simulink model "PushPullDCACConverter"  (R2018a)
settings: Solver=VariableStepAuto  StartTime=0.0  StopTime=0.3  RelTol=1e-3
libraries: powerlib x7, powerlib_meascontrol x1
settings Model: Creator=Rodney Tan  LastModifiedBy=Rodney Tan

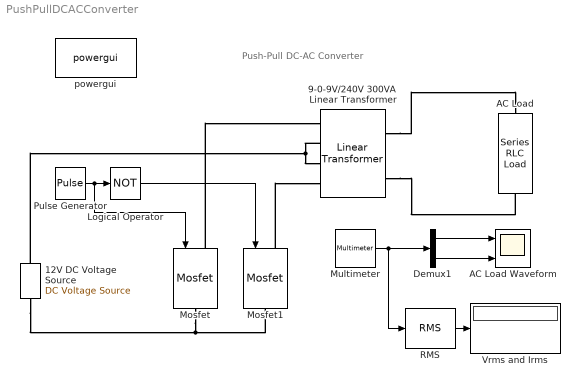
== system PushPullDCACConverter ==
  note: Push-Pull DC-AC Converter
  12V DC Voltage Source : powerlib/Electrical Sources/DC Voltage Source  Amplitude=12  Measurements=None
  9-0-9V/240V 300VA Linear Transformer : powerlib/Elements/Linear Transformer  UNITS=pu  NominalPower=[ 300 50 ]  winding1="[ 240  0.002  0.08 ]"  winding2="[ 9  0.002  0.08 ]"  ThreeWindings=on  winding3=[ 9 0.002 0.08 ]  RmLm=[ 500 500 ]  Measurements=None  DataType=off
  AC Load : powerlib/Elements/Series RLC Load  LConnTagsString=a  RConnTagsString=__new0  NominalVoltage=240  NominalFrequency=50  ActivePower=250  InductivePower=0  CapacitivePower=0  Setx0=off  InitialVoltage=0  SetiL0=off  InitialCurrent=0  Measurements=Branch voltage and current  LoadType=constant Z
  AC Load Waveform : Scope  NumInputPorts=2
  Demux1 : Demux  Outputs=2
  Logical Operator : Logic  Operator=NOT  AllPortsSameDT=off  OutDataTypeStr=boolean
  Mosfet : powerlib/Power Electronics/Mosfet  Ron=0.1  Lon=0  Rd=0.01  Vfd=0  IC=0  Rs=1e5  Cs=inf  Measurements=off
  Mosfet1 : powerlib/Power Electronics/Mosfet  Ron=0.1  Lon=0  Rd=0.01  Vfd=0  IC=0  Rs=1e5  Cs=inf  Measurements=off
  Multimeter : powerlib/Measurements/Multimeter  PhasorSimulation=off  OutputType=Complex  sel=[1 2]  L=2  Gain=[1 1]  yselected={'Ub: AC Load','Ib: AC Load'};  PSBOutputType=1  PSBequivalent=0  AxesSetting=[0,0.1,-100,100]  Display=0  SavedBlockNames=-11
  Pulse Generator : DiscretePulseGenerator  PulseType=Time based  Period=1/50  PulseWidth=50
  RMS : powerlib_meascontrol/Measurements/RMS  TrueRMS=on  Freq=50  RMSInit=0  Ts=0
  Vrms and Irms : Display
  powergui : powerlib/powergui  Priority=1  SimulationMode=Continuous  SampleTime=50e-6  frequency=60  Iterations=50  frequencyindice=0  Pbase=100e6  ErrMax=1e-4  UnitsV=kV  UnitsW=MW  buscounter=0  FunctionMessages=off  echomessages=off  EnableUseOfTLC=off  CurrentSourceSwitches=off  DisableSnubberDevices=off  DisableRonSwitches=off  DisableVfSwitches=off  DisplayEquations=off  SolverType=Tustin/Backward Euler (TBE)  Interpol=off  ExternalGateDelay=off  methode=off  Ts=100  x0status=blocks  SPID=on  SwTol=0  HookPort=off  RestoreLinks=warning  ResistiveCurrentMeasurement=off  Frange=[0:2:500]  Ylog=off  Xlog=on  ShowGrid=off  save=off  variable=ZData  structure=0  ZoomFFT=off  StartTime=0.0  cycles=1  DisplayStyle=1  fundamental=60  FreqAxis=off  MaxFrequency=1000  frequencyindicesteady=1  RmsSteady=1  display=off
  wires:
  Demux1/2 -> AC Load Waveform/2
  Demux1/1 -> AC Load Waveform/1
  RMS/1 -> Vrms and Irms/1
  Multimeter/1 -> Demux1/1, RMS/1
  Pulse Generator/1 -> Mosfet/1, Logical Operator/1
  Logical Operator/1 -> Mosfet1/1
  connections:
  Mosfet/LConn1 -- 9-0-9V/240V 300VA Linear Transformer/RConn1
  Mosfet1/LConn1 -- 9-0-9V/240V 300VA Linear Transformer/RConn4
  9-0-9V/240V 300VA Linear Transformer/RConn2 -- 12V DC Voltage Source/RConn1 -- 9-0-9V/240V 300VA Linear Transformer/RConn3
  Mosfet/RConn1 -- 12V DC Voltage Source/LConn1 -- Mosfet1/RConn1
  9-0-9V/240V 300VA Linear Transformer/LConn2 -- AC Load/RConn1
  9-0-9V/240V 300VA Linear Transformer/LConn1 -- AC Load/LConn1
